simulink model "sim_exp"  (Simulink 5.1)
settings: Solver=ode45  StartTime=0.0  StopTime=10.0  RelTol=1e-3
undefined symbols (not defined in the file or in its folder): sim_ref
libraries: mpt_sim x2
settings Model: Creator=michal  LastModifiedBy=kvasnica  ExtModeAutoUpdateStatusClock=off  SignalLoggingName=logsout  BooleanDataType=on  ProdHWDeviceType=Microprocessor  RTWOptions="-aEnforceIntegerDowncast=1 -aFoldNonRolledExpr=1 -aInlineInvariantSignals=0 -aInlineParameters=0 -aLocalBlockOutputs=1 -aRollThreshold=5 -aGenerateReport=0 -aGenCodeOnly=0 -aRTWVerbose=1 -aIncludeHyperlinkInReport=0 -aLaunchReport=0 -aForceParamTrailComments=0 -aGenerateComments=1 -aIgnoreCustomStorageClasses=1 -aIncHierarchyInIds=0 -aMaxRTWIdLen=31 -aShowEliminatedStatements=0 -aPrefixModelToSubsysFcnNames=1 -aIncDataTypeInIds=0 -aInsertBlockDesc=0 -aSimulinkBlockComments=1 -aInlinedPrmAccess=\"Literals\"  -aSuppressErrorStatus=0 -aModelReferenceCompliant=1 -aParenthesesLevel=\"Nominal\" -aSupportNonInlinedSFcns=1 -aSupportContinuousTime=1 -aSupportComplex=1 -aSupportNonFinite=1 -aSupportAbsoluteTime=1 -aTargetPreCompLibLocation=\"\" -aTargetLibSuffix=\"\" -aTargetFcnLib=\"ansi_tfl_tmw.mat\" -aMultiInstanceERTCode=0 -aLogVarNameModifier=\"rt_\" -aIsPILTarget=0 -aCombineOutputUpdateFcns=0 -aGenerateASAP2=0 -aGenerateTestInterfaces=0 -aGenerateSampleERTMain=0 -aGenerateFullHeader=1 -aUtilityFuncGeneration=\"Auto\" -aIncludeFileDelimiter=\"Auto\" -aIncludeMdlTerminateFcn=1 -aPurelyIntegerCode=0 -aERTCustomFileBanners=0 -aRTWCAPIStates=0 -aRTWCAPIParams=0 -aRTWCAPISignals=0 -aMatFileLogging=1 -aGenFloatMathFcnCalls=\"ANSI_C\" -aExtModeMexFile=\"ext_comm\" -aExtModeTransport=0 -aExtModeStaticAllocSize=1000000 -aExtModeTesting=0 -aExtModeStaticAlloc=0 -aExtMode=0"

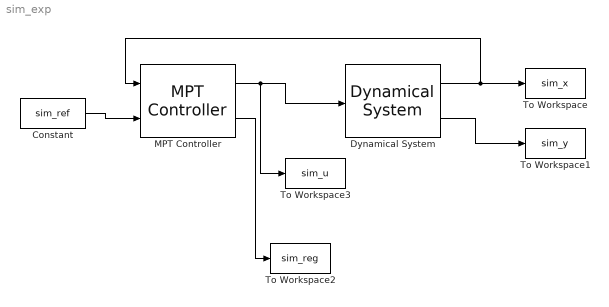
== system sim_exp ==
  Constant : Constant  Value=sim_ref
  Dynamical System : mpt_sim/Dynamical System  sysStruct=sim_sysStruct  x0=sim_x0  Ts=[]  constr=on
  MPT Controller : mpt_sim/MPT Controller  ctrl=sim_ctrl  Ts=[]  infbreak=on
  To Workspace : ToWorkspace  VariableName=sim_x  SampleTime=-1  SaveFormat=Array
  To Workspace1 : ToWorkspace  VariableName=sim_y  SampleTime=-1  SaveFormat=Array
  To Workspace2 : ToWorkspace  VariableName=sim_reg  SampleTime=-1  SaveFormat=Array
  To Workspace3 : ToWorkspace  VariableName=sim_u  SampleTime=-1  SaveFormat=Array
  wires:
  MPT Controller/1 -> Dynamical System/1, To Workspace3/1
  MPT Controller/2 -> To Workspace2/1
  Dynamical System/1 -> To Workspace/1, MPT Controller/1
  Dynamical System/2 -> To Workspace1/1
  Constant/1 -> MPT Controller/2
